simulink subsystem "Parking_ThorneFleissner"  (R2020b)
settings: Solver=VariableStepAuto  StartTime=0.0  StopTime=10.0  RelTol=1e-3
settings Model: Creator=rthom  LastModifiedBy=rthom

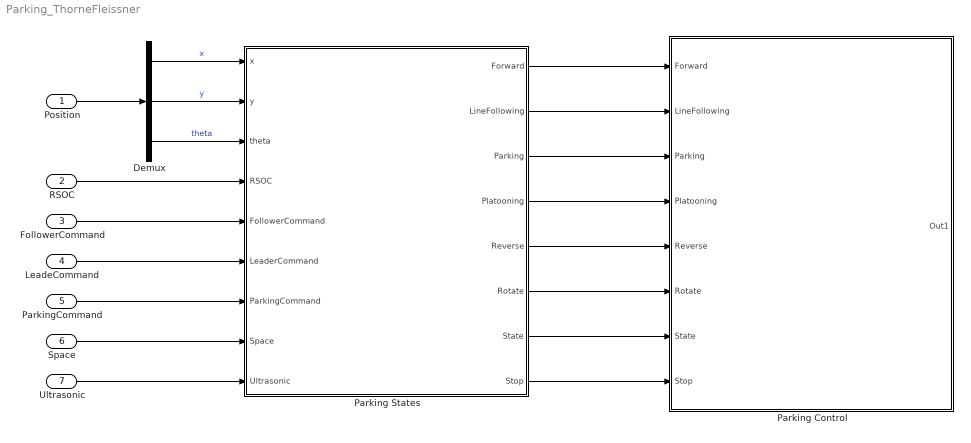
== system Parking_ThorneFleissner ==
  Position : Inport
  RSOC : Inport  Port=2
  FollowerCommand : Inport  Port=3
  LeadeCommand : Inport  Port=4
  ParkingCommand : Inport  Port=5
  Space : Inport  Port=6
  Ultrasonic : Inport  Port=7
  Demux : Demux  Outputs=3
  Parking Control : Subsystem
  Parking States : Stateflow chart  TreatAsAtomicUnit=on
  wires:
  Position/1 -> Demux/1
  Demux/2 -> Parking States/2(y)  "y"
  Demux/3 -> Parking States/3(theta)  "theta"
  Demux/1 -> Parking States/1(x)  "x"
  Parking States/1(Forward) -> Parking Control/1(Forward)
  Parking States/2(LineFollowing) -> Parking Control/2(LineFollowing)
  Parking States/3(Parking) -> Parking Control/3(Parking)
  Parking States/4(Platooning) -> Parking Control/4(Platooning)
  Parking States/5(Reverse) -> Parking Control/5(Reverse)
  Parking States/6(Rotate) -> Parking Control/6(Rotate)
  Parking States/7(State) -> Parking Control/7(State)
  Parking States/8(Stop) -> Parking Control/8(Stop)
  RSOC/1 -> Parking States/4(RSOC)
  FollowerCommand/1 -> Parking States/5(FollowerCommand)
  LeadeCommand/1 -> Parking States/6(LeaderCommand)
  Ultrasonic/1 -> Parking States/9(Ultrasonic)
  Space/1 -> Parking States/8(Space)
  ParkingCommand/1 -> Parking States/7(ParkingCommand)

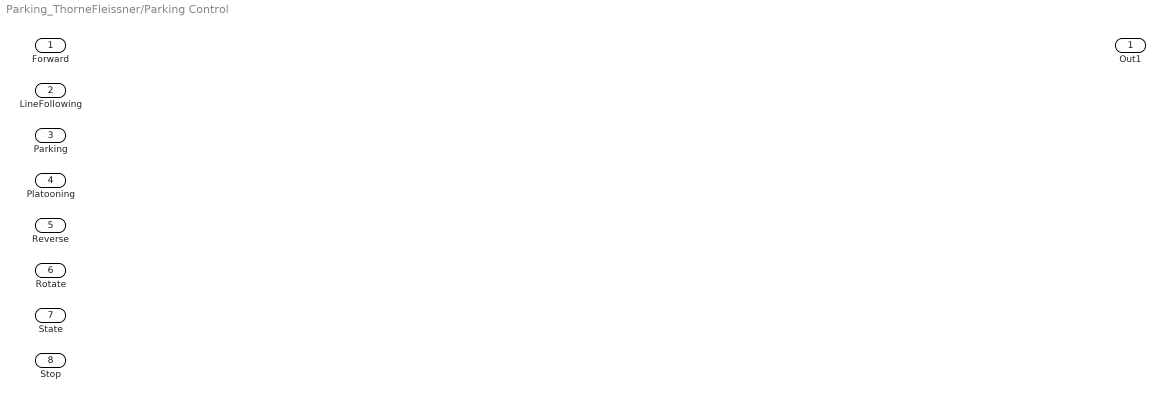
== system Parking_ThorneFleissner/Parking Control ==
  Forward : Inport
  LineFollowing : Inport  Port=2
  Parking : Inport  Port=3
  Platooning : Inport  Port=4
  Reverse : Inport  Port=5
  Rotate : Inport  Port=6
  State : Inport  Port=7
  Stop : Inport  Port=8
  Out1 : Outport

== stateflow chart Parking_ThorneFleissner/Parking States ==
  state IsLeader
    %EV is set as the leader
    entry:
    LineFollowing = 1;%Line Following enabled
    Platooning = 0;%Platooning disabled
    Stop = 0;%Stopping disabled
    Reverse = 0;%Reversing disabled
    Rotate = 0;%Rotating disabled
    Forward = 0;%Foward motion disabled
    Parking = 0;%Parking using ultrasonic sensor disabled
    State = 0;
  state IsFindingParking
    %EV rotates and moves toward parking position.
    entry:
    LineFollowing = 0;%Line Following disabled
    Platooning = 0;%Platooning disabled
    Stop = 0;%Stopping disabled
    Reverse = 0;%Reversing disabled
    Rotate = 1;%Rotate towards parking.
    Forward = 1;%Foward motion enabled
    Parking = 0;%Parking using ultrasonic sensor disabled
    State = 4;
  state IsParkingIntoSpace
    %EV rotates and moves toward parking position
    %using the ultrasonic sensor in parking mode.
    entry:
    LineFollowing = 0;%Line Following disabled
    Platooning = 0;%Platooning disabled
    Stop = 0;%Stopping disabled
    Reverse = 0;%Reversing disabled
    Rotate = 1;%Rotate perpendicular to the spot
    Forward = 1;%Foward motion enabled
    Parking = 1;%Parking using ultrasonic sensor enabled
    State = 5;
  state IsStopped
    %EV moves to the desired distance away from the
    %front of the parking space
    entry:
    LineFollowing = 0;%Line Following disabled
    Platooning = 0;%Platooning disabled
    Stop = 1;%Stopping enabled
    Reverse = 0;%Reversing disabled
    Rotate = 0;%Rotating disabled
    Forward = 0;%Foward motion disabled
    Parking = 0;%Parking using ultrasonic sensor disabled
    State = 6;
  state IsReversing
    %EV reverses out of parking spot and stages.
    entry:
    LineFollowing = 0;%Line Following disabled
    Platooning = 0;%Platooning disabled
    Stop = 0;%Stopping disabled
    Reverse = 1;%Reversing enabled
    Rotate = 0;%Rotating disabled
    Forward = 0;%Foward motion disabled
    Parking = 0;%Parking using ultrasonic sensor disabled
    State = 7;
  state IsReversed
    %EV rotates towards the lower portion of the track
    entry:
    LineFollowing = 0;%Line Following disabled
    Platooning = 0;%Platooning disabled
    Stop = 0;%Stopping disabled
    Reverse = 0;%Reversing disabled
    Rotate = -1;%Rotate -90 deg
    Forward = 0;%Foward motion disabled
    Parking = 0;%Parking using ultrasonic sensor disabled
    State = 8;
  state IsGoToStopSign
    %EV moves to the stop sign
    entry:
    LineFollowing = 0;%Line Following disabled
    Platooning = 0;%Platooning disabled
    Stop = 0;%Stopping disabled
    Reverse = 0;%Reversing disabled
    Rotate = 0;%Rotating disabled
    Forward = 1;%Foward motion enabled
    Parking = 0;%Parking using ultrasonic sensor disabled
    State = 9;
  state IsEnteringTrack
    %EV moves to the track entrance, enters track, and
    %rotates in the correct orientation.
    entry:
    LineFollowing = 0;%Line Following disabled
    Platooning = 0;%Platooning disabled
    Stop = 0;%Stopping disabled
    Reverse = 0;%Reversing disabled
    Rotate = -1;%Rotate -90 deg
    Forward = 1;%Foward motion enabled
    Parking = 0;%Parking using ultrasonic sensor disabled
    State = 10;
  state IsExitingTrack
    %EV reaches exit ramp and stops
    %using the line following and
    %platooning controllers, rotates
    %towards the parking area, then moves to staging .
    entry:
    LineFollowing = 0;%Line Following disabled
    Platooning = 0;%Platooning disabled
    Stop = 0;%Stopping disabled
    Reverse = 0;%Reverse disabled
    Rotate = -1;%Rotate enalbed, -90 deg
    Forward = 1;%Forward Motion off track enabled
    State = 3;
  state IsParking
    %EV is told to park and initializes
    %assocaited values. If the EV
    %reaches the ramp it moves to next
    %state. If parking button pressed
    %again, it will return to either leader
    %or follower state.
    entry:
    Stop = 0;%Stoping disabled
    Reverse = 0;%Reverse disabled
    Rotate = 0;%Rotate disabled
    State = 2;
  state IsFollower
    %EV is set as the follower
    entry:
    LineFollowing = 1;%Line Following enabled
    Platooning = 1;%Platooning enabled
    Stop = 0;%Stopping disabled
    Reverse = 0;%Reversing disabled
    Rotate = 0;%Rotating disabled
    Forward = 0;%Foward motion disabled
    Parking = 0;%Parking using ultrasonic sensor disabled
    State = 1;
  IsEnteringTrack -> IsLeader [order 1] : [LeaderCommand == 1 &&...
      | (x >= -0.5 && x <= -0.1) &&...
      | (y >= 0.3 && y <= 0.36)]
  (default) -> IsLeader
  IsParking -> IsLeader [order 2] : [ParkingCommand == 0 && ...
      | LeaderCommand ==1]
  IsLeader -> IsParking [order 2] : [ParkingCommand == 1]
  IsFollower -> IsLeader [order 1] : [LeaderCommand == 1]
  IsLeader -> IsFollower [order 1] : [FollowerCommand == 1]
  IsParking -> IsExitingTrack [order 1] : [(x <= 0.2 && x >= -0.2)...
      | && (y <= 3 && y >= 2)]
  IsStopped -> IsReversing : [RSOC == 100 ||...
      | ParkingCommand == 0]
  IsExitingTrack -> IsFindingParking : [(theta >= -93 && theta <= -87) &&...
      | ((Space == 3 && (x >= -0.3 && x <= 0.3) && (y >= 1.7 && y <= 1.9)) ||...
      | (Space == 2 &&  (x >= -0.3 && x <= 0.3) && (y >= 1.4 && y <= 1.6)) ||...
      | (Space == 1 &&  (x >= -0.3 && x <= 0.3) && (y >= 1.0 && y <= 1.2)))]
  IsFindingParking -> IsParkingIntoSpace : [((Space == 3 && (x >= -0.5 && x <= -0.4) && (y >= 1.5 && y <= 1.7)) ||...
      | (Space == 2 &&  (x >= -0.8 && x <= -0.7) && (y >= 1.1 && y <= 1.3)) ||...
      | (Space == 1 &&  (x >= -0.9 && x <= -0.8) && (y >= 0.7 && y <= 0.9)))]
  IsParkingIntoSpace -> IsStopped : [Ultrasonic <= 15]
  IsReversing -> IsReversed : [((Space == 3 && (x >= -0.3 && x <= 0.3) && (y >= 1.4 && y <= 1.9)) ||...
      | (Space == 2 &&  (x >= -0.3 && x <= 0.3) && (y >= 1.0 && y <= 1.3)) ||...
      | (Space == 1 &&  (x >= -0.3 && x <= 0.3) && (y >= 0.65 && y <= 0.1)))]
  IsReversed -> IsGoToStopSign : [theta >= -93 && theta <= -87]
  IsGoToStopSign -> IsEnteringTrack : [(x >= 0.017 & x <= 0.17) &&...
      | (y >= 0.45 && y <= 0.6)]
  IsFollower -> IsParking [order 2] : [ParkingCommand == 1]
  IsParking -> IsFollower [order 3] : [ParkingCommand == 0 && ...
      | FollowerCommand == 1]
  IsEnteringTrack -> IsFollower [order 2] : [FollowerCommand == 1 &&...
      | (x >= -0.5 && x <= -0.1) &&...
      | (y >= 0.3 && y <= 0.36)]
  data: x input; y input; theta input; RSOC input; FollowerCommand input; LeaderCommand input; ParkingCommand input; Space input; Ultrasonic input; Forward output; LineFollowing output; Parking output; Platooning output; Reverse output; Rotate output; State output; Stop output
